simulink model "RETRO_IFF_NON_LIN"  (R2022b)
settings: Solver=VariableStepAuto  StartTime=0.0  StopTime=28  RelTol=1e-3
model workspace (MATLAB code in the model file):
  | Kab=14;
  | Fa=4;
  | Kba=10;
  | Fb=4;
  | Kca=8;
  | Kcb=3.2;
  | Kcd=6;
  | Fc=2;
  | Kdc=6;
  | Fd=0.5;
  | Kia=5;
  | Fa=6;
  | In=0.3;
  | x_star=[0.25;0.625;0.0833;0];
settings Model: Creator=priya  LastModifiedBy=pxb271
settings SolverCC: AlgebraicLoopSolver=TrustRegion
settings DebuggingCC: UnconnectedInputMsg=warning  UnconnectedOutputMsg=warning  UnconnectedLineMsg=warning  SFMachineParentedDataDiag=warning
settings ModelReferenceCC: EnableRefExpFcnMdlSchedulingChecks=on
settings RTWCC: DLArmComputeVersion=19.05

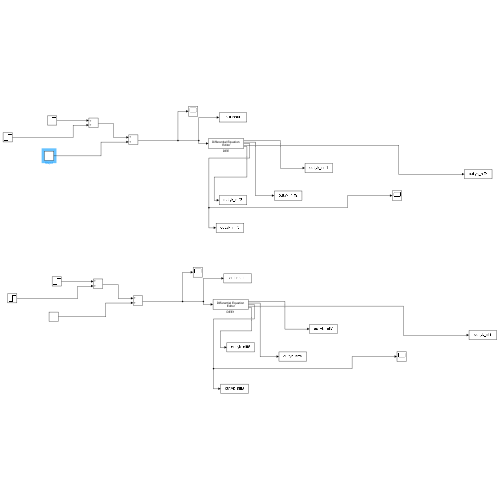
[thumbnail: Simulink's stored preview of the top-level diagram]
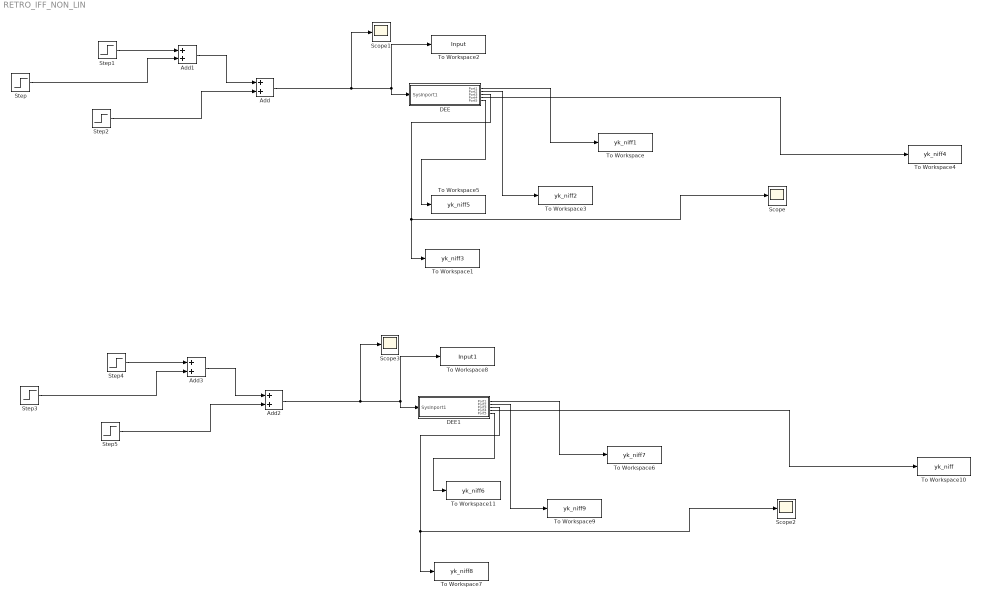
== system RETRO_IFF_NON_LIN ==
  Add{,1..3} (4 alike) : Sum
  DEE : Subsystem  mask(Differential Equation Editor (DEE)){}
      settings: OpenFcn=diffeqed
      mask Display: disp('Differential Equation\n Editor')
  DEE1 : Subsystem  mask(Differential Equation Editor (DEE)){}
      settings: OpenFcn=diffeqed
      mask Display: disp('Differential Equation\n Editor')
  Scope{,1..3} (4 alike) : Scope
  Step : Step  Time=10  After=30  SampleTime=0
  Step1 : Step  Time=0  After=15  SampleTime=0
  Step2 : Step  Time=20  After=40  SampleTime=0
  Step3 : Step  Time=10  After=30  SampleTime=0
  Step4 : Step  Time=0  After=15  SampleTime=0
  Step5 : Step  Time=20  After=40  SampleTime=0
  To Workspace : ToWorkspace  VariableName=yk_niff1  SampleTime=-1
  To Workspace1 : ToWorkspace  VariableName=yk_niff3  SampleTime=-1
  To Workspace10 : ToWorkspace  VariableName=yk_niff  SampleTime=-1
  To Workspace11 : ToWorkspace  VariableName=yk_niff6  SampleTime=-1
  To Workspace2 : ToWorkspace  VariableName=Input  SampleTime=-1
  To Workspace3 : ToWorkspace  VariableName=yk_niff2  SampleTime=-1
  To Workspace4 : ToWorkspace  VariableName=yk_niff4  SampleTime=-1
  To Workspace5 : ToWorkspace  VariableName=yk_niff5  SampleTime=-1
  To Workspace6 : ToWorkspace  VariableName=yk_niff7  SampleTime=-1
  To Workspace7 : ToWorkspace  VariableName=yk_niff8  SampleTime=-1
  To Workspace8 : ToWorkspace  VariableName=Input1  SampleTime=-1
  To Workspace9 : ToWorkspace  VariableName=yk_niff9  SampleTime=-1
  wires:
  Step1/1 -> Add1/1
  Step/1 -> Add1/2
  Step2/1 -> Add/2
  Add1/1 -> Add/1
  Add/1 -> To Workspace2/1, DEE/1(SysInport1), Scope1/1
  DEE/1(Port1) -> To Workspace/1
  DEE/2(Port2) -> To Workspace3/1
  DEE/3(Port3) -> Scope/1, To Workspace1/1
  DEE/4(Port4) -> To Workspace4/1
  DEE/5(Port5) -> To Workspace5/1
  DEE1/3(Port3) -> Scope2/1, To Workspace7/1
  Add2/1 -> To Workspace8/1, DEE1/1(SysInport1), Scope3/1
  DEE1/1(Port1) -> To Workspace6/1
  DEE1/2(Port2) -> To Workspace9/1
  Step5/1 -> Add2/2
  Step3/1 -> Add3/2
  Add3/1 -> Add2/1
  Step4/1 -> Add3/1
  DEE1/4(Port4) -> To Workspace10/1
  DEE1/5(Port5) -> To Workspace11/1

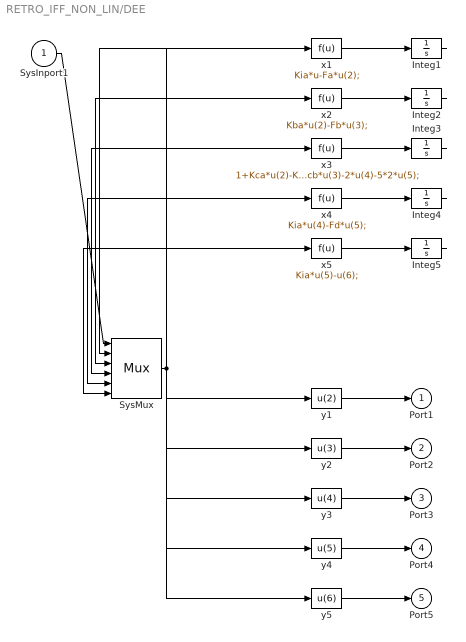
== system RETRO_IFF_NON_LIN/DEE ==
  SysInport1 : Inport
  Integ1 : Integrator  InitialCondition=x_star(1)
  Integ2 : Integrator  InitialCondition=x_star(2)
  Integ3 : Integrator  InitialCondition=0.25
  Integ4 : Integrator  InitialCondition=x_star(4)
  Integ5 : Integrator
  SysMux : Mux  Inputs=6
  x1 : Fcn  Expr=Kia*u-Fa*u(2);
  x2 : Fcn  Expr=Kba*u(2)-Fb*u(3);
  x3 : Fcn  Expr=1+Kca*u(2)-Kcb*u(3)-2*u(4)-5*2*u(5);
  x4 : Fcn  Expr=Kia*u(4)-Fd*u(5);
  x5 : Fcn  Expr=Kia*u(5)-u(6);
  y1 : Fcn  Expr=u(2)
  y2 : Fcn  Expr=u(3)
  y3 : Fcn  Expr=u(4)
  y4 : Fcn  Expr=u(5)
  y5 : Fcn  Expr=u(6)
  Port1 : Outport
  Port2 : Outport  Port=2
  Port3 : Outport  Port=3
  Port4 : Outport  Port=4
  Port5 : Outport  Port=5
  wires:
  SysInport1/1 -> SysMux/1
  SysMux/1 -> x1/1, x2/1, x3/1, x4/1, x5/1, y1/1, y2/1, y3/1, y4/1, y5/1
  x1/1 -> Integ1/1
  Integ1/1 -> SysMux/2
  x2/1 -> Integ2/1
  Integ2/1 -> SysMux/3
  x3/1 -> Integ3/1
  Integ3/1 -> SysMux/4
  x4/1 -> Integ4/1
  Integ4/1 -> SysMux/5
  x5/1 -> Integ5/1
  Integ5/1 -> SysMux/6
  y1/1 -> Port1/1
  y2/1 -> Port2/1
  y3/1 -> Port3/1
  y4/1 -> Port4/1
  y5/1 -> Port5/1

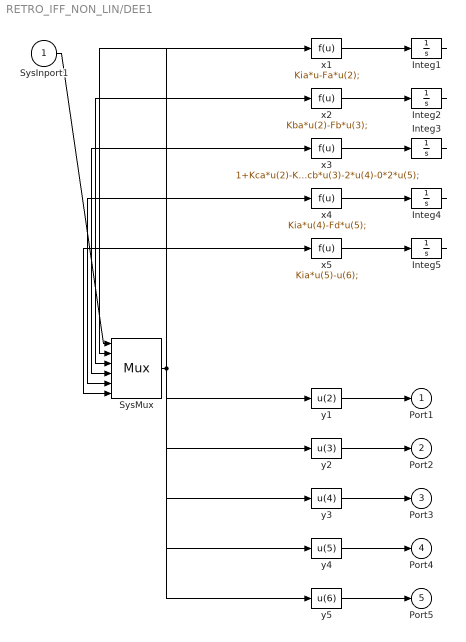
== system RETRO_IFF_NON_LIN/DEE1 ==
  SysInport1 : Inport
  Integ1 : Integrator  InitialCondition=x_star(1)
  Integ2 : Integrator  InitialCondition=x_star(2)
  Integ3 : Integrator  InitialCondition=0.25
  Integ4 : Integrator  InitialCondition=x_star(4)
  Integ5 : Integrator
  SysMux : Mux  Inputs=6
  x1 : Fcn  Expr=Kia*u-Fa*u(2);
  x2 : Fcn  Expr=Kba*u(2)-Fb*u(3);
  x3 : Fcn  Expr=1+Kca*u(2)-Kcb*u(3)-2*u(4)-0*2*u(5);
  x4 : Fcn  Expr=Kia*u(4)-Fd*u(5);
  x5 : Fcn  Expr=Kia*u(5)-u(6);
  y1 : Fcn  Expr=u(2)
  y2 : Fcn  Expr=u(3)
  y3 : Fcn  Expr=u(4)
  y4 : Fcn  Expr=u(5)
  y5 : Fcn  Expr=u(6)
  Port1 : Outport
  Port2 : Outport  Port=2
  Port3 : Outport  Port=3
  Port4 : Outport  Port=4
  Port5 : Outport  Port=5
  wires:
  SysInport1/1 -> SysMux/1
  SysMux/1 -> x1/1, x2/1, x3/1, x4/1, x5/1, y1/1, y2/1, y3/1, y4/1, y5/1
  x1/1 -> Integ1/1
  Integ1/1 -> SysMux/2
  x2/1 -> Integ2/1
  Integ2/1 -> SysMux/3
  x3/1 -> Integ3/1
  Integ3/1 -> SysMux/4
  x4/1 -> Integ4/1
  Integ4/1 -> SysMux/5
  x5/1 -> Integ5/1
  Integ5/1 -> SysMux/6
  y1/1 -> Port1/1
  y2/1 -> Port2/1
  y3/1 -> Port3/1
  y4/1 -> Port4/1
  y5/1 -> Port5/1
